simulink library "AeroLib"  (Simulink 6.0)
settings: Solver=ode45  SolverMode=SingleTasking  StartTime=0.0  StopTime=10.0  RelTol=1e-3
undefined symbols (not defined in the file): Aero, Ap, Atm, Control, Controls, Eng, Flight_cg, Flight_DamperON, Flight_delta_isa, Flight_DeltaSpiral, Flight_InertiaSelect, Flight_ixx, Flight_ixz, Flight_iyy, Flight_izz, Flight_latitude, Flight_LoiterLenght, Flight_LoiterMode, Flight_LoiterRadius, Flight_longitude, Flight_MaxTargetPoints, Flight_SensorsON, Flight_TimeStep, Flight_TowerWind_X, Flight_TowerWind_Y, Flight_TowerWind_Z, Flight_TowerWindON, Flight_Trimming, Flight_TurbON, Flight_weight, Flight_WindGustON, Flight_WindShearON, Flight_ycg, Flight_zcg, Geom, Lgear, Mass, PEG_CDwbnp, PEG_CLht, PEG_CLht_elev, PEG_CLwbnp, PEG_CMht, PEG_CMwbnp, PEG_CNbeta, PEG_CNr, PEG_CNrud, PEG_CRail, PEG_CRbeta, PEG_CRp, PEG_CRrud, PEG_CYbeta, PEG_CYrud, pow, Sensors
libraries: AeroLib x133, simulink3 x49, simulink x37, aerospace x11
(part 7 of 7)

== system AeroLib/Autopilot/Autopilot/Dampers/Pitch_Damper/Limit_Alpha_and_Speed ==
  TAS : Inport  Port=1  LatchInput=off
  Reset : Inport  Port=2  LatchInput=off
  From_Prop : Inport  Port=3  LatchInput=off
  Alpha : Inport  Port=4  LatchInput=off
  From_Inputs : Inport  Port=5  LatchInput=off
  Alpha Limit : Subsystem
  Bus Selector1 : BusSelector  DialogController=Simulink.DDGSource_Bus  OutputSignals=StopBooster
  Bus Selector2 : BusSelector  DialogController=Simulink.DDGSource_Bus  OutputSignals=IRU_TAS_kt
  Bus Selector3 : BusSelector  DialogController=Simulink.DDGSource_Bus  OutputSignals=BoosterON
  Logical Operator : Logic  Operator=OR
  Logical Operator1 : Logic  Operator=NOT
  Product1 : Product  SaturateOnIntegerOverflow=on  InputSameDT=on
  Saturation : Saturate  UpperLimit=5  LowerLimit=-5
  Speed_Limit : Subsystem
  Sum : Sum  Inputs=|++  SaturateOnIntegerOverflow=on  InputSameDT=on
  Elev_minSpeed : Outport
  wires:
  Saturation/1 -> Elev_minSpeed/1
  From_Prop/1 -> Bus Selector1/1
  Speed_Limit/1(Elev) -> Product1/1
  TAS/1 -> Bus Selector2/1
  Reset/1 -> Speed_Limit/2(Reset_In), Alpha Limit/2(Reset_In)
  Product1/1 -> Sum/1
  Alpha/1 -> Alpha Limit/1(Alpha)
  Alpha Limit/1(Elev) -> Sum/2
  Bus Selector2/1 -> Speed_Limit/1(TAS)  "<IRU_TAS_kt>"
  Sum/1 -> Saturation/1
  From_Inputs/1 -> Bus Selector3/1
  Bus Selector3/1 -> Logical Operator1/1  "<BoosterON>"
  Bus Selector1/1 -> Logical Operator/1  "<StopBooster>"
  Logical Operator1/1 -> Logical Operator/2
  Logical Operator/1 -> Product1/2

== system AeroLib/Autopilot/Autopilot/Dampers/Pitch_Damper/Pitch_damp ==
  From_INS : Inport  Port=1  LatchInput=off
  Bus Selector : BusSelector  DialogController=Simulink.DDGSource_Bus  OutputSignals=IRU_Q_degps,FSC_VD_mps
  Gain1 : Gain  Gain=Kq  SaturateOnIntegerOverflow=on
  Gain4 : Gain  Gain=Kd  SaturateOnIntegerOverflow=on
  Sum : Sum  SaturateOnIntegerOverflow=on  InputSameDT=on
  Elev_cmd : Outport
  wires:
  Gain4/1 -> Sum/2
  Bus Selector/2 -> Gain4/1  "<FSC_VD_mps>"
  Bus Selector/1 -> Gain1/1  "<IRU_Q_degps>"
  From_INS/1 -> Bus Selector/1
  Sum/1 -> Elev_cmd/1
  Gain1/1 -> Sum/1

== system AeroLib/Autopilot/Autopilot/Dampers/Roll_Damper/Phi Limit ==
  Reset_In : Inport  Port=1  LatchInput=off
  Phi : Inport  Port=2  LatchInput=off
  Abs : Abs  SaturateOnIntegerOverflow=on
  Bus Selector : BusSelector  DialogController=Simulink.DDGSource_Bus  OutputSignals=IRU_Phi_deg
  Constant : Constant  Value=0
  Gain : Gain  Gain=0.1  SaturateOnIntegerOverflow=on
  Stateless_HighPass : AeroLib/AMS_StatelessFilters/Stateless_HighPass
  Subsystem : Subsystem
  Sum2 : Sum  Inputs=|-+  SaturateOnIntegerOverflow=on  InputSameDT=on
  Switch : Switch  Threshold=Ap.Track.LimPhi+1  SaturateOnIntegerOverflow=on  InputSameDT=on
  Tau : Constant  Value=0.1
  Ail : Outport
  wires:
  Switch/1 -> Ail/1
  Subsystem/1(Ail_Com) -> Sum2/2
  Constant/1 -> Switch/3
  Bus Selector/1 -> Abs/1, Subsystem/1(Phi), Stateless_HighPass/2  "<IRU_Phi_deg>"
  Abs/1 -> Switch/2
  Gain/1 -> Sum2/1
  Sum2/1 -> Switch/1
  Stateless_HighPass/1 -> Gain/1
  Reset_In/1 -> Stateless_HighPass/1
  Tau/1 -> Stateless_HighPass/3
  Phi/1 -> Bus Selector/1

== system AeroLib/Autopilot/Autopilot/Dampers/Roll_Damper/Roll_damp ==
  From_Sen : Inport  Port=1  LatchInput=off
  Reset_In : Inport  Port=2  LatchInput=off
  Bus Selector : BusSelector  DialogController=Simulink.DDGSource_Bus  OutputSignals=IRU_P_degps,FSC_TrackMag_deg
  Damph_Gain : Gain  Gain=Kp  SaturateOnIntegerOverflow=on
  Damph_Gain1 : Gain  Gain=Kd  SaturateOnIntegerOverflow=on
  Deriv_Limit : Subsystem
  Stateless_HighPass : AeroLib/AMS_StatelessFilters/Stateless_HighPass
  Sum : Sum  SaturateOnIntegerOverflow=on  InputSameDT=on
  Tau : Constant  Value=0.1
  Ail_cmd : Outport
  wires:
  Deriv_Limit/1(Out) -> Damph_Gain1/1
  Sum/1 -> Ail_cmd/1
  Stateless_HighPass/1 -> Deriv_Limit/1(In)
  Damph_Gain1/1 -> Sum/2
  From_Sen/1 -> Bus Selector/1
  Bus Selector/1 -> Damph_Gain/1  "<IRU_P_degps>"
  Bus Selector/2 -> Stateless_HighPass/2  "<FSC_TrackMag_deg>"
  Damph_Gain/1 -> Sum/1
  Reset_In/1 -> Stateless_HighPass/1
  Tau/1 -> Stateless_HighPass/3

== system AeroLib/Autopilot/Autopilot/Dampers/Yaw_Damper/PID_Ny ==
  Err : Inport  Port=1  LatchInput=off
  From_Reset : Inport  Port=2  LatchInput=off
  IntGain : Gain  Gain=I  SaturateOnIntegerOverflow=on
  PID_Prop_Gamma : Gain  Gain=P  SaturateOnIntegerOverflow=on
  Stateless_HighPass : AeroLib/AMS_StatelessFilters/Stateless_HighPass
  Stateless_Integrator1 : AeroLib/AMS_StatelessFilters/Stateless_Integrator
  Sum : Sum  Inputs=+++  SaturateOnIntegerOverflow=on  InputSameDT=on
  Tau : Constant  Value=0.1
  Xo : Constant  Value=0
  Cmd : Outport  InitialOutput=0
  wires:
  Sum/1 -> Cmd/1
  Stateless_Integrator1/1 -> IntGain/1
  IntGain/1 -> Sum/2
  PID_Prop_Gamma/1 -> Sum/1
  Stateless_HighPass/1 -> Sum/3
  Err/1 -> Stateless_Integrator1/3, Stateless_HighPass/2, PID_Prop_Gamma/1
  Xo/1 -> Stateless_Integrator1/2
  From_Reset/1 -> Stateless_Integrator1/1, Stateless_HighPass/1
  Tau/1 -> Stateless_HighPass/3

== system AeroLib/Autopilot/Autopilot/Guidance/Loiter_modes/Last_point_data ==
  From_Sensors : Inport  Port=1  LatchInput=off
  Target_N : Inport  Port=2  LatchInput=off
  Bus Selector1 : BusSelector  DialogController=Simulink.DDGSource_Bus  OutputSignals=FSC_TrackMag_deg,FSC_Xdist_m,FSC_Ydist_m
  Demux : Demux  Outputs=3
  Fcn1 : Fcn  Expr=u(1) - u(2) == 1
  Mem : Memory  X0=[0 0 0]
  Memory : Memory
  Mux : Mux  Inputs=2
  Mux1 : Mux  Inputs=3
  Sw4 : Switch  Threshold=0.5  SaturateOnIntegerOverflow=on  InputSameDT=on
  deg-->rad : Gain  Gain=pi/180  SaturateOnIntegerOverflow=on
  LastX_m : Outport
  LastY_m : Outport  Port=2
  LastTrack_rad : Outport  Port=3
  wires:
  Demux/3 -> LastY_m/1
  Demux/2 -> LastX_m/1
  Demux/1 -> deg-->rad/1
  Mux1/1 -> Sw4/1
  Bus Selector1/3 -> Mux1/3  "<FSC_Ydist_m>"
  Bus Selector1/2 -> Mux1/2  "<FSC_Xdist_m>"
  Bus Selector1/1 -> Mux1/1  "<FSC_TrackMag_deg>"
  Target_N/1 -> Mux/1, Memory/1
  From_Sensors/1 -> Bus Selector1/1
  deg-->rad/1 -> LastTrack_rad/1
  Sw4/1 -> Mem/1
  Fcn1/1 -> Sw4/2
  Mem/1 -> Demux/1, Sw4/3
  Memory/1 -> Mux/2
  Mux/1 -> Fcn1/1

== system AeroLib/Autopilot/Autopilot/Guidance/Loiter_modes/Serpentine_Loiter_mode ==
  From_FSC : Inport  Port=1  LatchInput=off
  X_last : Inport  Port=2  LatchInput=off
  Y_last : Inport  Port=3  LatchInput=off
  Track_last : Inport  Port=4  LatchInput=off
  From_Reset : Inport  Port=5  LatchInput=off
  Bus Selector2 : BusSelector  DialogController=Simulink.DDGSource_Bus  OutputSignals=IRU_TAS_kt
  Constant : Constant
  Constant1 : Constant
  Counter_Point : AeroLib/Autopilot/Counter_Point  MinDist=Ap.Loiter.MinDist
  Fcn3 : Fcn  Expr=u+1
  Look-Up Table : Lookup  DialogController=Simulink.DDGSource  InputValues=[-360 -270 -180-eps -180+eps -90 0 90 180-eps 180+eps 270 360]  OutputValues=[0 90 180 -180 -90 0 90 180 -180 -90 0]  SaturateOnIntegerOverflow=on
  Memory_Dist : Memory  X0=1000000000
  Target_Errors : AeroLib/Autopilot/Target_Errors
  Terminator{,1..3} (4 alike) : Terminator
  Turn_Radius : Subsystem
  coord_serpent_or_lazy8 : Subsystem
  kt-->mps : Gain  Gain=0.5144444  SaturateOnIntegerOverflow=on
  Track_Err : Outport
  Point_N : Outport  Port=2
  wires:
  Turn_Radius/1(Track_Err) -> Track_Err/1
  Look-Up Table/1 -> Turn_Radius/1(Track_Error)
  coord_serpent_or_lazy8/2(X_target_m) -> Target_Errors/2
  coord_serpent_or_lazy8/1(Y_target_m) -> Target_Errors/1
  From_Reset/1 -> Counter_Point/2
  kt-->mps/1 -> Turn_Radius/2(TAS_mps)
  From_FSC/1 -> Bus Selector2/1, Target_Errors/4
  Y_last/1 -> coord_serpent_or_lazy8/3(Y_last)
  X_last/1 -> coord_serpent_or_lazy8/2(X_last)
  Track_last/1 -> coord_serpent_or_lazy8/1(track_last)
  Bus Selector2/1 -> kt-->mps/1  "<IRU_TAS_kt>"
  Target_Errors/3 -> Look-Up Table/1
  Counter_Point/1 -> Fcn3/1
  Memory_Dist/1 -> Counter_Point/1
  Fcn3/1 -> Point_N/1, coord_serpent_or_lazy8/4(Point_N)
  Target_Errors/2 -> Terminator/1
  Target_Errors/4 -> Terminator1/1
  Target_Errors/5 -> Terminator2/1
  Target_Errors/6 -> Terminator3/1
  Target_Errors/1 -> Memory_Dist/1
  Constant/1 -> Target_Errors/3
  Constant1/1 -> Target_Errors/5

== system AeroLib/Autopilot/Autopilot/Guidance/Loiter_modes/Spiral_and_circle_Loiter_mode ==
  LastTrack : Inport  Port=1  LatchInput=off
  From_FSC : Inport  Port=2  LatchInput=off
  From_Reset : Inport  Port=3  LatchInput=off
  Enable : EnablePort
  Bus Selector1 : BusSelector  DialogController=Simulink.DDGSource_Bus  OutputSignals=IRU_TAS_kt
  Bus Selector2 : BusSelector  DialogController=Simulink.DDGSource_Bus  OutputSignals=FSC_TrackMag_deg
  Constant2 : Constant  Orientation=left  Value=Flight_LoiterRadius
  Constant3 : Constant  Orientation=left  Value=Flight_DeltaSpiral
  Counter_Point : AeroLib/Autopilot/Counter_Point  MinDist=0.25
  Fcn1 : Fcn  Expr=abs( abs(u) - 90 )
  Fcn2 : Fcn  Orientation=left  Expr=u(2) + u(3)*u(1)
  Loiter_BankAngle : Fcn  Expr=atan(u(2)^2/(Atm.grav*u(1)))*180/pi/Ap.Track.err
  Mux1 : Mux  Orientation=left  Inputs=3
  Mux2 : Mux  Inputs=2
  Sum1 : Sum  Inputs=-+|  SaturateOnIntegerOverflow=on  InputSameDT=on
  kt-->mps : Gain  Gain=0.5144444  SaturateOnIntegerOverflow=on
  rad->deg : Gain  Gain=180/pi  SaturateOnIntegerOverflow=on
  Track_Err : Outport
  Point_N : Outport  Port=2
  wires:
  From_Reset/1 -> Counter_Point/2
  Constant3/1 -> Mux1/3
  Constant2/1 -> Mux1/2
  Mux1/1 -> Fcn2/1
  LastTrack/1 -> rad->deg/1
  Counter_Point/1 -> Mux1/1, Point_N/1
  Fcn2/1 -> Mux2/1
  kt-->mps/1 -> Mux2/2
  Bus Selector1/1 -> kt-->mps/1  "<IRU_TAS_kt>"
  Sum1/1 -> Fcn1/1
  Bus Selector2/1 -> Sum1/2  "<FSC_TrackMag_deg>"
  Loiter_BankAngle/1 -> Track_Err/1
  Mux2/1 -> Loiter_BankAngle/1
  From_FSC/1 -> Bus Selector1/1, Bus Selector2/1
  rad->deg/1 -> Sum1/1
  Fcn1/1 -> Counter_Point/1

== system AeroLib/Autopilot/Autopilot/Guidance/Loiter_modes/Subsystem ==
  Target_N : Inport  Port=1  LatchInput=off
  Constant1 : Constant  Value=Flight_LoiterMode
  Constant2 : Constant  Value=Flight_MaxTargetPoints
  Fcn1 : Fcn  Expr=u == 1
  Fcn2 : Fcn  Expr=u(1) >u(2)+0.5
  Logical Operator1 : Logic
  Mux : Mux  Inputs=2
  Enable_com : Outport
  wires:
  Target_N/1 -> Mux/1
  Constant2/1 -> Mux/2
  Mux/1 -> Fcn2/1
  Fcn1/1 -> Logical Operator1/2
  Constant1/1 -> Fcn1/1
  Logical Operator1/1 -> Enable_com/1
  Fcn2/1 -> Logical Operator1/1

== system AeroLib/Autopilot/Autopilot/Guidance/Target_Errors/AP_RATO ==
  FromSensor : Inport  Port=1  LatchInput=off
  From_Prop : Inport  Port=2  LatchInput=off
  From_Inputs : Inport  Port=3  LatchInput=off
  Bus Selector : BusSelector  DialogController=Simulink.DDGSource_Bus  OutputSignals=StopBooster
  Bus Selector1 : BusSelector  DialogController=Simulink.DDGSource_Bus  OutputSignals=IRU_TAS_kt,FSC_Altitude_ft
  Bus Selector2 : BusSelector  DialogController=Simulink.DDGSource_Bus  OutputSignals=BoosterON
  Fcn : Fcn  Expr=u(1) >= Ap.Booster.Vmin && u(2) >= Ap.Booster.Altmin
  Fcn1 : Fcn  Expr=1-u
  Mux2 : Mux  Inputs=2
  Product1 : Product  SaturateOnIntegerOverflow=on  InputSameDT=on
  Sum : Sum  Inputs=|++  SaturateOnIntegerOverflow=on  InputSameDT=on
  HoldAlt_ON : Outport
  wires:
  Fcn/1 -> Product1/2
  Bus Selector/1 -> Product1/1  "<StopBooster>"
  Bus Selector1/1 -> Mux2/1  "<IRU_TAS_kt>"
  Bus Selector1/2 -> Mux2/2  "<FSC_Altitude_ft>"
  Mux2/1 -> Fcn/1
  FromSensor/1 -> Bus Selector1/1
  From_Prop/1 -> Bus Selector/1
  From_Inputs/1 -> Bus Selector2/1
  Bus Selector2/1 -> Fcn1/1  "<BoosterON>"
  Product1/1 -> Sum/1
  Sum/1 -> HoldAlt_ON/1
  Fcn1/1 -> Sum/2

== system AeroLib/EquationsOfMotion/Equations_of_Motion/EQM Six-DOF/Geodetic_Frame_EQM/Longitude_Bound ==
  note: Latitude
      |
      | Longitude
  Lat Lon : Inport  Port=1  LatchInput=off
  Demux : Demux  Outputs=2
  Fcn2 : Fcn  Expr=u(1) + 360*u(2)
  Fcn3 : Fcn  Expr=u(1) - 360*u(2)
  Mux : Mux  Inputs=2
  Mux1 : Mux  Inputs=2
  Poles : Subsystem
  Subsystem : Subsystem
  Subsystem1 : Subsystem
  Switch2 : Switch  Threshold=-180  SaturateOnIntegerOverflow=on  InputSameDT=on
  Switch3 : Switch  Threshold=180  SaturateOnIntegerOverflow=on  InputSameDT=on
  Lon_deg : Outport
  Lat_deg : Outport  Port=2
  wires:
  Subsystem1/1(Out1) -> Mux1/2
  Mux1/1 -> Fcn2/1
  Subsystem/1(Out1) -> Mux/2
  Mux/1 -> Fcn3/1
  Lat Lon/1 -> Demux/1
  Demux/2 -> Poles/2(Longitude_deg)
  Demux/1 -> Lat_deg/1, Poles/1(Latitude_deg)
  Fcn2/1 -> Switch2/3
  Fcn3/1 -> Switch3/1
  Switch2/1 -> Switch3/2, Subsystem/1(In1), Mux/1, Switch3/3
  Switch3/1 -> Lon_deg/1
  Poles/1(LimLongitude_deg) -> Switch2/1, Subsystem1/1(In1), Mux1/1, Switch2/2

== system AeroLib/EquationsOfMotion/Equations_of_Motion/EQM Six-DOF/Geodetic_Frame_EQM/WGS 84 ==
  Latitude_rad : Inport  Port=1  LatchInput=off
  Altitude_m : Inport  Port=2  LatchInput=off
  Fcn : Fcn  Expr=(6378137+ u(2) )*(1-0.00669438)/(u(1)^1.5)
  Fcn1 : Fcn  Expr=(6378137+ u(2) )/sqrt(u(1))
  Fcn2 : Fcn  Expr=1-0.00669437999*(sin(u(1)))^2
  Fcn3 : Fcn  Expr=6378137 - 21385*sin(u(1))+u(2)
  Mux2 : Mux  Inputs=2
  Mux3 : Mux  Inputs=2
  RadOfCurv_ver_m : Outport
  GeogHight_m : Outport  Port=2
  RadOfCurv_mer_m : Outport  Port=3
  wires:
  Altitude_m/1 -> Mux2/2, Mux3/2
  Mux2/1 -> Fcn3/1
  Mux3/1 -> Fcn1/1, Fcn/1
  Latitude_rad/1 -> Mux2/1, Fcn2/1
  Fcn3/1 -> GeogHight_m/1
  Fcn1/1 -> RadOfCurv_ver_m/1
  Fcn/1 -> RadOfCurv_mer_m/1
  Fcn2/1 -> Mux3/1

== system AeroLib/EquationsOfMotion/Equations_of_Motion/EQM Six-DOF/Geodetic_Frame_EQM/Zero-->Eps ==
  In1 : Inport  Port=1  LatchInput=off
  Constant1 : Constant  Value=eps
  Fcn2 : Fcn  Expr=abs(u) > eps
  Product : Product  SaturateOnIntegerOverflow=on  InputSameDT=on
  Sign : Signum
  Switch : Switch  Threshold=0.5  SaturateOnIntegerOverflow=on  InputSameDT=on
  Out1 : Outport
  wires:
  Fcn2/1 -> Switch/2
  Sign/1 -> Product/1
  Constant1/1 -> Product/2
  Product/1 -> Switch/3
  Switch/1 -> Out1/1
  In1/1 -> Fcn2/1, Sign/1, Switch/1

== system AeroLib/EquationsOfMotion/Equations_of_Motion/EQM Six-DOF/Quaternion_Euler/Euler ==
  P Q R : Inport  Port=1  LatchInput=off
  Enable : EnablePort
  EQM Euler_Angles : Subsystem
  PHIang THETAang PSIang : Integrator
  Euler_Trim : Outport  InitialOutput=0
  wires:
  EQM Euler_Angles/1(phidot thetadot psidot) -> PHIang THETAang PSIang/1
  PHIang THETAang PSIang/1 -> EQM Euler_Angles/2(phi theta psi), Euler_Trim/1
  P Q R/1 -> EQM Euler_Angles/1(p q r)

== system AeroLib/EquationsOfMotion/Equations_of_Motion/EQM Six-DOF/Quaternion_Euler/Quaternion_Comp ==
  Flight_q : Inport  Port=1  LatchInput=off
  P Q R : Inport  Port=2  LatchInput=off
  Enable : EnablePort
  DeadZone : DeadZone  LowerValue=-eps  UpperValue=eps  SaturateOnIntegerOverflow=on
  QUA2EUL : AeroLib/CoordinateSystems/QUA2EUL
  Quaternion Normalize : Subsystem  mask(Quaternion Normalize){}
      mask help: qout = q/sqrt(q(1)^2+q(2)^2+q(3)^2+q(4)^2)
      mask init:
      | pos = get_param(gcb, 'Position');
      | width = pos(3) - pos(1); height = pos(4) - pos(2);
      | fontsize = get_param(gcb, 'fontsize');
      | scale=fontsize/10;
  Quaternion Derivative : Subsystem
      mask Display: disp('q = q1 + i*q2 + j*q3 + k*q4\n---------------------------------------------\nq1dot =-0.5*(q2*P + q3*Q + q4*R)\nq2dot = 0.5*(q1*P + q3*R -  q4*Q)\nq3dot = 0.5*(q1*Q + q3*P - q2*R)\nq4dot = 0.5*(q1*R + q2*Q - q3*P)')
  q1 q2 q3 q4 : Integrator  InitialConditionSource=external
  Euler  angles : Outport
  Quaternion : Outport  Port=2
  wires:
  DeadZone/1 -> q1 q2 q3 q4/1
  Quaternion Normalize/1(qnorm) -> QUA2EUL/1, Quaternion Derivative/2(q), Quaternion/1  "q1 q2 q3 q4"
  Flight_q/1 -> q1 q2 q3 q4/2
  Quaternion Derivative/1(q_dot) -> DeadZone/1
  q1 q2 q3 q4/1 -> Quaternion Normalize/1(q)
  P Q R/1 -> Quaternion Derivative/1(p q r)
  QUA2EUL/1 -> Euler  angles/1

== system AeroLib/EquationsOfMotion/Equations_of_Motion/EQM_Outputs/Inertilal Positions/Accelerations ==
  DCM : Inport  Port=1  LatchInput=off
  AG_b : Inport  Port=2  LatchInput=off
  Demux1 : Demux  Outputs=3
  Product : Product  Multiplication=Matrix(*)  SaturateOnIntegerOverflow=on  InputSameDT=on
  Xacc : Outport
  Yacc : Outport  Port=2
  Zacc : Outport  Port=3
  wires:
  Demux1/3 -> Zacc/1  "Zacc"
  Demux1/2 -> Yacc/1  "Yacc"
  Demux1/1 -> Xacc/1  "Xacc"
  AG_b/1 -> Product/2
  Product/1 -> Demux1/1  "AccI"
  DCM/1 -> Product/1

== system AeroLib/EquationsOfMotion/Equations_of_Motion/EQM_Outputs/Inertilal Positions/FlightPathVel ==
  AlongTrackAcc : Inport  Port=1  LatchInput=off
  Ang_rad : Inport  Port=2  LatchInput=off
  Zacc : Inport  Port=3  LatchInput=off
  Mux : Mux
  Trigonometric Function : Trigonometry
  Trigonometric Function1 : Trigonometry  Operator=cos
  Vert_acc : Fcn  Expr=- u / Atm.grav
  XcosA - YsinA : Fcn  Expr=(u(3)*u(2) - u(4)*u(1)) / Atm.grav
  AlongPathAcc_g : Outport
  VertAcc_g : Outport  Port=2
  wires:
  Vert_acc/1 -> VertAcc_g/1
  XcosA - YsinA/1 -> AlongPathAcc_g/1
  Mux/1 -> XcosA - YsinA/1
  Trigonometric Function/1 -> Mux/1
  Trigonometric Function1/1 -> Mux/2
  Zacc/1 -> Vert_acc/1, Mux/4
  AlongTrackAcc/1 -> Mux/3
  Ang_rad/1 -> Trigonometric Function1/1, Trigonometric Function/1

== system AeroLib/EquationsOfMotion/Equations_of_Motion/EQM_Outputs/Inertilal Positions/HeadingAcc ==
  Xacc : Inport  Port=1  LatchInput=off
  Yacc : Inport  Port=2  LatchInput=off
  Ang_rad : Inport  Port=3  LatchInput=off
  Mux : Mux
  Trigonometric Function : Trigonometry
  Trigonometric Function1 : Trigonometry  Operator=cos
  XcosA - YsinA : Fcn  Expr=(u(3)*u(2) - u(4)*u(1)) / Atm.grav
  YcosA + XsinA : Fcn  Expr=(u(4)*u(2) + u(3)*u(1)) / Atm.grav
  Along : Outport
  Cross : Outport  Port=2
  wires:
  YcosA + XsinA/1 -> Cross/1
  XcosA - YsinA/1 -> Along/1
  Mux/1 -> YcosA + XsinA/1, XcosA - YsinA/1
  Trigonometric Function/1 -> Mux/1
  Trigonometric Function1/1 -> Mux/2
  Yacc/1 -> Mux/4
  Xacc/1 -> Mux/3
  Ang_rad/1 -> Trigonometric Function1/1, Trigonometric Function/1

== system AeroLib/EquationsOfMotion/Equations_of_Motion/EQM_Outputs/Inertilal Positions/Positions ==
  Xe : Inport  Port=1  LatchInput=off
  Demux : Demux  Outputs=3
  Ground_Height : Constant  Value=0
  Sum : Sum  Inputs=|--  SaturateOnIntegerOverflow=on  InputSameDT=on
  m_to_ft : Gain  Gain=3.28083  SaturateOnIntegerOverflow=on
  Xdist : Outport  InitialOutput=0
  Ydist : Outport  Port=2  InitialOutput=0
  Hagl_m : Outport  Port=3  InitialOutput=0
  Hagl_ft : Outport  Port=4  InitialOutput=0
  wires:
  m_to_ft/1 -> Hagl_ft/1
  Sum/1 -> m_to_ft/1, Hagl_m/1
  Xe/1 -> Demux/1
  Demux/3 -> Sum/1
  Ground_Height/1 -> Sum/2
  Demux/2 -> Ydist/1
  Demux/1 -> Xdist/1

== system AeroLib/EquationsOfMotion/Equations_of_Motion/EQM_Outputs/Inertilal Positions/TrackAcc ==
  Ang_rad : Inport  Port=1  LatchInput=off
  Xdot : Inport  Port=2  LatchInput=off
  Ydot : Inport  Port=3  LatchInput=off
  Xacc : Inport  Port=4  LatchInput=off
  Yacc : Inport  Port=5  LatchInput=off
  Mux : Mux  Inputs=6
  Trigonometric Function : Trigonometry
  Trigonometric Function1 : Trigonometry  Operator=cos
  XcosA - YsinA : Fcn  Expr=(u(3)*u(2) - u(4)*u(1))
  YcosA + XsinA : Fcn  Expr=(u(4)*u(2) + u(3)*u(1))
  YcosA + XsinA1 : Fcn  Expr=(u(6)*u(2) + u(5)*u(1))
  AlongAcc : Outport
  CrossAcc : Outport  Port=2
  CrossTrackVel : Outport  Port=3
  wires:
  YcosA + XsinA1/1 -> CrossTrackVel/1
  Ydot/1 -> Mux/6
  Xdot/1 -> Mux/5
  YcosA + XsinA/1 -> CrossAcc/1
  XcosA - YsinA/1 -> AlongAcc/1
  Mux/1 -> YcosA + XsinA1/1, YcosA + XsinA/1, XcosA - YsinA/1
  Trigonometric Function/1 -> Mux/1
  Trigonometric Function1/1 -> Mux/2
  Yacc/1 -> Mux/4
  Xacc/1 -> Mux/3
  Ang_rad/1 -> Trigonometric Function1/1, Trigonometric Function/1

== system AeroLib/EquationsOfMotion/Equations_of_Motion/EQM_Outputs/Inertilal Positions/Velocities ==
  Vi : Inport  Port=1  LatchInput=off
  Fcn : Fcn  Expr=sqrt(u(1)*u(1)+u(2)*u(2))
  Fcn1 : Fcn  Expr=-u(3)
  Fcn2 : Fcn  Expr=u(1)
  Fcn3 : Fcn  Expr=-atan2(u(3),u(4))
  Fcn4 : Fcn  Expr=atan2(u(2),u(1))
  Fcn5 : Fcn  Expr=u(2)
  Mux1 : Mux  Inputs=2
  m/s_to_kt : Gain  Gain=1.943844  SaturateOnIntegerOverflow=on
  m/s_to_kt3 : Gain  Gain=196.8504  SaturateOnIntegerOverflow=on
  rad_to_deg : Gain  Gain=57.29578  SaturateOnIntegerOverflow=on
  rad_to_deg1 : Gain  Gain=57.29578  SaturateOnIntegerOverflow=on
  Hdot_mps : Outport  InitialOutput=0
  GroundSpeed_kt : Outport  Port=2  InitialOutput=0
  Gamma_deg : Outport  Port=3  InitialOutput=0
  Track_deg : Outport  Port=4  InitialOutput=0
  Hdot_ftpmin : Outport  Port=5  InitialOutput=0
  Track_rad : Outport  Port=6
  Xdot_mps : Outport  Port=7
  Ydot_mps : Outport  Port=8
  Gamma_rad : Outport  Port=9
  wires:
  Fcn3/1 -> rad_to_deg/1, Gamma_rad/1
  m/s_to_kt3/1 -> Hdot_ftpmin/1
  Fcn5/1 -> Ydot_mps/1
  Fcn2/1 -> Xdot_mps/1
  rad_to_deg1/1 -> Track_deg/1
  rad_to_deg/1 -> Gamma_deg/1
  m/s_to_kt/1 -> GroundSpeed_kt/1
  Fcn1/1 -> Hdot_mps/1, m/s_to_kt3/1
  Mux1/1 -> Fcn5/1, Fcn2/1, Fcn1/1, Fcn4/1, Fcn3/1
  Fcn/1 -> m/s_to_kt/1, Mux1/2  "GNS"
  Vi/1 -> Mux1/1, Fcn/1  "Ve"
  Fcn4/1 -> rad_to_deg1/1, Track_rad/1

== system AeroLib/GroundReactions/Landing_Gear/GHM Ground_Reactions/Reactions1/Inertial2Body ==
  FgLMG_I : Inport  Port=1  LatchInput=off
  FgNG_I : Inport  Port=2  LatchInput=off
  FgRMG_I : Inport  Port=3  LatchInput=off
  EulerRad : Inport  Port=4  LatchInput=off
  Demux : Demux  Outputs=3
  Ground2Body_LMG : Subsystem
  Ground2Body_NG : Subsystem
  Ground2Body_RMG : Subsystem
  Sum : Sum  Inputs=3  SaturateOnIntegerOverflow=on  InputSameDT=on
  Terminator : Terminator
  cos : Trigonometry  Operator=cos
  cos1 : Trigonometry  Operator=cos
  sin : Trigonometry
  sin1 : Trigonometry
  Fg_B : Outport
  FgLMG_B : Outport  Port=2
  FgNG_B : Outport  Port=3
  FgRMG_B : Outport  Port=4
  wires:
  Sum/1 -> Fg_B/1
  Ground2Body_RMG/1(Fg_B) -> Sum/3, FgRMG_B/1
  Ground2Body_NG/1(Fg_B) -> Sum/2, FgNG_B/1
  Ground2Body_LMG/1(Fg_B) -> Sum/1, FgLMG_B/1
  FgNG_I/1 -> Ground2Body_NG/1(Fb_I)
  FgLMG_I/1 -> Ground2Body_LMG/1(Fb_I)
  FgRMG_I/1 -> Ground2Body_RMG/1(Fb_I)
  cos/1 -> Ground2Body_NG/3(CosPhi), Ground2Body_LMG/3(CosPhi), Ground2Body_RMG/3(CosPhi)
  sin/1 -> Ground2Body_NG/2(SinPhi), Ground2Body_LMG/2(SinPhi), Ground2Body_RMG/2(SinPhi)
  cos1/1 -> Ground2Body_NG/5(CosThe), Ground2Body_LMG/5(CosThe), Ground2Body_RMG/5(CosThe)
  sin1/1 -> Ground2Body_NG/4(SinThe), Ground2Body_LMG/4(SinThe), Ground2Body_RMG/4(SinThe)
  Demux/3 -> Terminator/1  "psi"
  Demux/2 -> cos1/1, sin1/1  "theta"
  Demux/1 -> cos/1, sin/1  "phi"
  EulerRad/1 -> Demux/1

== system AeroLib/GroundReactions/Landing_Gear/GHM Ground_Reactions/Reactions1/NoseGearForces ==
  MUeNg : Inport  Port=1  LatchInput=off
  MUsNg : Inport  Port=2  LatchInput=off
  FstrNg : Inport  Port=3  LatchInput=off
  NoseWheelAng : Inport  Port=4  LatchInput=off
  Fcn : Fcn  Expr=u(3)*u(1) - u(4)*u(2)
  Fcn1 : Fcn  Expr=u(4)*u(1) + u(3)*u(2)
  Gain2 : Gain  Gain=-1  SaturateOnIntegerOverflow=on
  Mux : Mux
  Mux1 : Mux  Inputs=3
  Product1 : Product  SaturateOnIntegerOverflow=on  InputSameDT=on
  Product2 : Product  SaturateOnIntegerOverflow=on  InputSameDT=on
  Trigonometric Function : Trigonometry  Operator=cos
  Trigonometric Function1 : Trigonometry
  deg_to_rad : Gain  Gain=pi/180  SaturateOnIntegerOverflow=on
  FgearNG : Outport
  wires:
  NoseWheelAng/1 -> deg_to_rad/1
  Product1/1 -> Mux1/1
  Fcn/1 -> Product1/1  "Vx"
  Gain2/1 -> FgearNG/1
  FstrNg/1 -> Mux1/3, Product1/2, Product2/2
  Fcn1/1 -> Product2/1  "Vy"
  Product2/1 -> Mux1/2
  Mux/1 -> Fcn1/1, Fcn/1
  MUsNg/1 -> Mux/4
  MUeNg/1 -> Mux/3
  Trigonometric Function1/1 -> Mux/2
  Trigonometric Function/1 -> Mux/1
  Mux1/1 -> Gain2/1
  deg_to_rad/1 -> Trigonometric Function/1, Trigonometric Function1/1

== system AeroLib/GroundReactions/Landing_Gear/Left Main Gear Dynamics/Ground_Tire Friction/Friction Coeff ==
  Brake : Inport  Port=1  PortDimensions=1  LatchInput=off
  Ug : Inport  Port=2  PortDimensions=1  LatchInput=off
  Vg : Inport  Port=3  PortDimensions=1  LatchInput=off
  TireForce : Inport  Port=4  PortDimensions=1  LatchInput=off
  Constant : Constant  Value=.018
  Constant1 : Constant  Value=0.001
  Constant2 : Constant  Value=0.93
  Cpower : Constant  Value=110
  Fcn : Fcn  Expr=atan2(u(1),u(2))*180/pi
  Fcn2 : Fcn  Expr=2*u
  Fcn3 : Fcn  Expr=0.67-.0003*u
  Fcn4 : Fcn  Expr=u(3)+(u(1)-u(3))*u(2)
  MinMax1 : MinMax  Function=max  Inputs=2  SaturateOnIntegerOverflow=on  InputSameDT=on
  Mux : Mux  Inputs=2
  Mux2 : Mux  Inputs=3
  Product : Product  Inputs=**//  SaturateOnIntegerOverflow=on  InputSameDT=on
  Product1 : Product  SaturateOnIntegerOverflow=on  InputSameDT=on
  Saturation : Saturate  UpperLimit=1000  LowerLimit=1
  Sign : Signum
  MUside : Outport
  MUeff : Outport  Port=2
  wires:
  Mux/1 -> Fcn/1
  Vg/1 -> Mux/1
  Ug/1 -> Saturation/1, Sign/1
  Saturation/1 -> Mux/2, Fcn3/1
  TireForce/1 -> MinMax1/2
  Fcn/1 -> Product/2  "Beta"
  Constant2/1 -> Product/3
  MinMax1/1 -> Product/4
  Product/1 -> MUside/1  "MUside"
  Fcn3/1 -> Mux2/1  "MUdry"
  Brake/1 -> Mux2/2
  Mux2/1 -> Fcn4/1
  Constant/1 -> Mux2/3  "MuRoll"
  Constant1/1 -> MinMax1/1
  Cpower/1 -> Fcn2/1
  Fcn2/1 -> Product/1
  Fcn4/1 -> Product1/2
  Sign/1 -> Product1/1
  Product1/1 -> MUeff/1

== system AeroLib/GroundReactions/Landing_Gear/Nose Gear Dynamics/Ground_Tire Friction/Friction Coeff ==
  Ug : Inport  Port=1  PortDimensions=1  LatchInput=off
  Vg : Inport  Port=2  PortDimensions=1  LatchInput=off
  TireForce : Inport  Port=3  PortDimensions=1  LatchInput=off
  Constant1 : Constant  Value=0.001
  Constant2 : Constant  Value=0.93
  Constant4 : Constant  Value=.018
  Cpower : Constant  Value=110
  Fcn : Fcn  Expr=atan2(u(1),u(2))*180/pi
  Fcn2 : Fcn  Expr=2*u
  MinMax1 : MinMax  Function=max  Inputs=2  SaturateOnIntegerOverflow=on  InputSameDT=on
  Mux : Mux  Inputs=2
  Product : Product  Inputs=**//  SaturateOnIntegerOverflow=on  InputSameDT=on
  Product2 : Product  SaturateOnIntegerOverflow=on  InputSameDT=on
  Saturation : Saturate  UpperLimit=1000  LowerLimit=1
  Sign1 : Signum
  MUside : Outport
  MUeff : Outport  Port=2
  wires:
  Product2/1 -> MUeff/1
  Fcn2/1 -> Product/1
  Cpower/1 -> Fcn2/1
  Constant1/1 -> MinMax1/1
  Product/1 -> MUside/1  "MUside"
  MinMax1/1 -> Product/4
  Constant2/1 -> Product/3
  Fcn/1 -> Product/2  "Beta"
  TireForce/1 -> MinMax1/2
  Saturation/1 -> Mux/2
  Ug/1 -> Saturation/1, Sign1/1
  Vg/1 -> Mux/1
  Mux/1 -> Fcn/1
  Sign1/1 -> Product2/1
  Constant4/1 -> Product2/2  "MuRoll"

== system AeroLib/GroundReactions/Landing_Gear/Right Main Gear Dynamics/Ground_Tire Friction/Friction Coeff ==
  Brake : Inport  Port=1  PortDimensions=1  LatchInput=off
  Ug : Inport  Port=2  PortDimensions=1  LatchInput=off
  Vg : Inport  Port=3  PortDimensions=1  LatchInput=off
  TireForce : Inport  Port=4  PortDimensions=1  LatchInput=off
  Constant : Constant  Value=.018
  Constant1 : Constant  Value=0.001
  Constant2 : Constant  Value=0.93
  Cpower : Constant  Value=110
  Fcn : Fcn  Expr=atan2(u(1),u(2))*180/pi
  Fcn2 : Fcn  Expr=2*u
  Fcn3 : Fcn  Expr=0.67-.0003*u
  Fcn4 : Fcn  Expr=u(3)+(u(1)-u(3))*u(2)
  MinMax1 : MinMax  Function=max  Inputs=2  SaturateOnIntegerOverflow=on  InputSameDT=on
  Mux : Mux  Inputs=2
  Mux2 : Mux  Inputs=3
  Product : Product  Inputs=**//  SaturateOnIntegerOverflow=on  InputSameDT=on
  Product1 : Product  SaturateOnIntegerOverflow=on  InputSameDT=on
  Saturation : Saturate  UpperLimit=1000  LowerLimit=1
  Sign : Signum
  MUside : Outport
  MUeff : Outport  Port=2
  wires:
  Mux/1 -> Fcn/1
  Vg/1 -> Mux/1
  Ug/1 -> Saturation/1, Sign/1
  Saturation/1 -> Mux/2, Fcn3/1
  TireForce/1 -> MinMax1/2
  Fcn/1 -> Product/2  "Beta"
  Constant2/1 -> Product/3
  MinMax1/1 -> Product/4
  Product/1 -> MUside/1  "MUside"
  Fcn3/1 -> Mux2/1  "MUdry"
  Brake/1 -> Mux2/2
  Mux2/1 -> Fcn4/1
  Constant/1 -> Mux2/3  "MuRoll"
  Constant1/1 -> MinMax1/1
  Cpower/1 -> Fcn2/1
  Fcn2/1 -> Product/1
  Fcn4/1 -> Product1/2
  Sign/1 -> Product1/1
  Product1/1 -> MUeff/1

== system AeroLib/Sensors/Inertial_Reference_Unit/Accelerometers/Sensors/SensorsOFF ==
  Clock : Clock
      settings: Decimation=10
  Constant1 : Constant  Value=Flight_SensorsON
  Fcn : Fcn  Expr=u <= 0+eps
  or : Logic  Operator=OR
  or1 : Logic  Operator=NOT
  SensorsOFF : Outport
  wires:
  or1/1 -> or/1
  or/1 -> SensorsOFF/1
  Fcn/1 -> or/2
  Constant1/1 -> or1/1  "DT"
  Clock/1 -> Fcn/1

== system AeroLib/Autopilot/Autopilot/Dampers/Pitch_Damper/Limit_Alpha_and_Speed/Alpha Limit ==
  Alpha : Inport  Port=1  LatchInput=off
  Reset_In : Inport  Port=2  LatchInput=off
  Constant : Constant  Value=0
  Fcn : Fcn  Expr=-(u-Ap.Alt.MinAlpha)
  Gain2 : Gain  Gain=1.2  SaturateOnIntegerOverflow=on
  Stateless_HighPass1 : AeroLib/AMS_StatelessFilters/Stateless_HighPass
  Sum2 : Sum  Inputs=|-+  SaturateOnIntegerOverflow=on  InputSameDT=on
  Switch : Switch  Threshold=Ap.Alt.MinAlpha  SaturateOnIntegerOverflow=on  InputSameDT=on
  Tau : Constant  Value=0.1
  Elev : Outport
  wires:
  Tau/1 -> Stateless_HighPass1/3
  Reset_In/1 -> Stateless_HighPass1/1
  Switch/1 -> Elev/1
  Gain2/1 -> Sum2/1
  Fcn/1 -> Sum2/2
  Sum2/1 -> Switch/1
  Constant/1 -> Switch/3
  Alpha/1 -> Switch/2, Fcn/1, Stateless_HighPass1/2
  Stateless_HighPass1/1 -> Gain2/1

== system AeroLib/Autopilot/Autopilot/Dampers/Pitch_Damper/Limit_Alpha_and_Speed/Speed_Limit ==
  TAS : Inport  Port=1  LatchInput=off
  Reset_In : Inport  Port=2  LatchInput=off
  Constant : Constant  Value=0
  Fcn : Fcn  Expr=-(u-Ap.Alt.Vmin)
  Gain1 : Gain  Gain=-8  SaturateOnIntegerOverflow=on
  Gain2 : Gain  Gain=1.2  SaturateOnIntegerOverflow=on
  Stateless_HighPass : AeroLib/AMS_StatelessFilters/Stateless_HighPass
  Sum2 : Sum  Inputs=|-+  SaturateOnIntegerOverflow=on  InputSameDT=on
  Switch : Switch  Threshold=Ap.Alt.Vmin  SaturateOnIntegerOverflow=on  InputSameDT=on
  Tau : Constant  Value=0.1
  Elev : Outport
  wires:
  Gain1/1 -> Elev/1
  Sum2/1 -> Switch/3
  Constant/1 -> Switch/1
  Stateless_HighPass/1 -> Gain2/1
  TAS/1 -> Switch/2, Fcn/1, Stateless_HighPass/2
  Fcn/1 -> Sum2/2
  Gain2/1 -> Sum2/1
  Switch/1 -> Gain1/1
  Reset_In/1 -> Stateless_HighPass/1
  Tau/1 -> Stateless_HighPass/3

== system AeroLib/Autopilot/Autopilot/Dampers/Roll_Damper/Phi Limit/Subsystem ==
  Phi : Inport  Port=1  LatchInput=off
  Fcn1 : Fcn  Expr=u >= 0
  Fcn2 : Fcn  Expr=-( u - Ap.Track.LimPhi)*0.4
  Fcn3 : Fcn  Expr=-( u + Ap.Track.LimPhi)*0.4
  Switch1 : Switch  Threshold=0.5  SaturateOnIntegerOverflow=on  InputSameDT=on
  Ail_Com : Outport
  wires:
  Switch1/1 -> Ail_Com/1
  Phi/1 -> Fcn1/1, Fcn3/1, Fcn2/1
  Fcn3/1 -> Switch1/3
  Fcn2/1 -> Switch1/1
  Fcn1/1 -> Switch1/2

== system AeroLib/Autopilot/Autopilot/Dampers/Roll_Damper/Roll_damp/Deriv_Limit ==
  In : Inport  Port=1  LatchInput=off
  Constant1 : Constant  Value=Flight_TimeStep
  Mux : Mux  Inputs=2
  Product : Product  SaturateOnIntegerOverflow=on  InputSameDT=on
  limit : Fcn  Expr=abs(u(1)) < 15*u(2)
  Out : Outport
  wires:
  In/1 -> Product/1, Mux/1
  Product/1 -> Out/1
  limit/1 -> Product/2
  Mux/1 -> limit/1
  Constant1/1 -> Mux/2

== system AeroLib/Autopilot/Autopilot/Guidance/Loiter_modes/Serpentine_Loiter_mode/Turn_Radius ==
  Track_Error : Inport  Port=1  LatchInput=off
  TAS_mps : Inport  Port=2  LatchInput=off
  Abs : Abs  SaturateOnIntegerOverflow=on
  Constant : Constant  Value=Flight_LoiterRadius
  Fcn1 : Fcn  Expr=abs(u(1)) < abs(u(2))*1.1
  Loiter_BankAngle : Fcn  Expr=atan(u(2)^2/(Atm.grav*u(1)))*180/pi/Ap.Track.err
  Mux2 : Mux  Inputs=2
  Mux3 : Mux  Inputs=2
  Product : Product  SaturateOnIntegerOverflow=on  InputSameDT=on
  Sign : Signum
  Switch : Switch  Threshold=0.5  SaturateOnIntegerOverflow=on  InputSameDT=on
  Track_Err : Outport
  wires:
  TAS_mps/1 -> Mux2/2
  Constant/1 -> Mux2/1
  Product/1 -> Switch/3
  Sign/1 -> Product/1
  Abs/1 -> Mux3/2, Product/2
  Loiter_BankAngle/1 -> Abs/1
  Switch/1 -> Track_Err/1
  Mux3/1 -> Fcn1/1
  Fcn1/1 -> Switch/2
  Mux2/1 -> Loiter_BankAngle/1
  Track_Error/1 -> Mux3/1, Sign/1, Switch/1

== system AeroLib/Autopilot/Autopilot/Guidance/Loiter_modes/Serpentine_Loiter_mode/coord_serpent_or_lazy8 ==
  track_last : Inport  Port=1  LatchInput=off
  X_last : Inport  Port=2  LatchInput=off
  Y_last : Inport  Port=3  LatchInput=off
  Point_N : Inport  Port=4  LatchInput=off
  Constant1 : Constant  Value=Flight_LoiterMode
  Demux : Demux  Outputs=2
  Gain1 : Gain  Gain=-1  SaturateOnIntegerOverflow=on
  LazyEight_Coor : Subsystem
  Mux1 : Mux  Inputs=2
  Product : Product  Multiplication=Matrix(*)  SaturateOnIntegerOverflow=on  InputSameDT=on
  Reshape : simulink/Math Operations/Reshape  OutputDimensionality=Row vector  OutputDimensions=[1,1]
  Serpentine_Coor : Subsystem
  Sum : Sum  Inputs=|++  SaturateOnIntegerOverflow=on  InputSameDT=on
  Switch : Switch  Threshold=2.5  SaturateOnIntegerOverflow=on  InputSameDT=on
  turn_transform : Subsystem
  Y_target_m : Outport
  X_target_m : Outport  Port=2
  wires:
  Constant1/1 -> Switch/2
  LazyEight_Coor/1(XY) -> Switch/1
  Switch/1 -> Reshape/1
  Serpentine_Coor/1(XY) -> Switch/3
  Gain1/1 -> turn_transform/1(Track_rad)
  Reshape/1 -> Product/1
  turn_transform/1(MatrixTransform) -> Product/2
  Y_last/1 -> Mux1/2
  X_last/1 -> Mux1/1
  Demux/2 -> Y_target_m/1
  Demux/1 -> X_target_m/1
  track_last/1 -> Gain1/1
  Sum/1 -> Demux/1
  Point_N/1 -> Serpentine_Coor/1(Point_N), LazyEight_Coor/1(Point_N)
  Product/1 -> Sum/1
  Mux1/1 -> Sum/2

== system AeroLib/EquationsOfMotion/Equations_of_Motion/EQM Six-DOF/Geodetic_Frame_EQM/Longitude_Bound/Poles ==
  Latitude_deg : Inport  Port=1  LatchInput=off
  Longitude_deg : Inport  Port=2  LatchInput=off
  Fcn1 : Fcn  Expr=abs(abs(u ) - 90) < 0.00001
  Fcn2 : Fcn  Expr=u(1)+180*u(2)
  Memory : Memory
  Mux : Mux  Inputs=2
  Sum : Sum  Inputs=|++  SaturateOnIntegerOverflow=on  InputSameDT=on
  Switch2 : Switch  Threshold=0.5  SaturateOnIntegerOverflow=on  InputSameDT=on
  LimLongitude_deg : Outport
  wires:
  Mux/1 -> Fcn2/1
  Fcn2/1 -> Switch2/1
  Fcn1/1 -> Sum/1
  Sum/1 -> Memory/1
  Memory/1 -> Sum/2, Switch2/2, Mux/2
  Longitude_deg/1 -> Switch2/3, Mux/1
  Switch2/1 -> LimLongitude_deg/1
  Latitude_deg/1 -> Fcn1/1

== system AeroLib/EquationsOfMotion/Equations_of_Motion/EQM Six-DOF/Geodetic_Frame_EQM/Longitude_Bound/Subsystem ==
  In1 : Inport  Port=1  LatchInput=off
  Constant : Constant
  Fcn1 : Fcn  Expr=u/360
  MinMax : MinMax  Function=max  Inputs=2  SaturateOnIntegerOverflow=on  InputSameDT=on
  Rounding Function : Rounding  Operator=round
  Out1 : Outport
  wires:
  Rounding Function/1 -> Out1/1
  In1/1 -> Fcn1/1
  Fcn1/1 -> MinMax/1
  MinMax/1 -> Rounding Function/1
  Constant/1 -> MinMax/2

== system AeroLib/EquationsOfMotion/Equations_of_Motion/EQM Six-DOF/Geodetic_Frame_EQM/Longitude_Bound/Subsystem1 ==
  In1 : Inport  Port=1  LatchInput=off
  Constant : Constant
  Fcn1 : Fcn  Expr=abs(u/360)
  MinMax : MinMax  Function=max  Inputs=2  SaturateOnIntegerOverflow=on  InputSameDT=on
  Rounding Function : Rounding  Operator=round
  Out1 : Outport
  wires:
  Constant/1 -> MinMax/2
  MinMax/1 -> Rounding Function/1
  Fcn1/1 -> MinMax/1
  In1/1 -> Fcn1/1
  Rounding Function/1 -> Out1/1

== system AeroLib/EquationsOfMotion/Equations_of_Motion/EQM Six-DOF/Quaternion_Euler/Euler/EQM Euler_Angles ==
  p q r : Inport  Port=1  LatchInput=off
  phi theta psi : Inport  Port=2  LatchInput=off
  Mux1 : Mux  Inputs=[3 3]
  Mux2 : Mux  Inputs=3
  phidot : Fcn  Expr=u[1]+u[2]*sin(u[4])*tan(u[5])+u[3]*cos(u[4])*tan(u[5])
  psidot : Fcn  Expr=u[2]*sin(u[4])/cos(u[5])+u[3]*cos(u[4])/cos(u[5])
  thetadot : Fcn  Expr=u[2]*cos(u[4])-u[3]*sin(u[4])
  phidot thetadot psidot : Outport  InitialOutput=0
  wires:
  phidot/1 -> Mux2/1
  thetadot/1 -> Mux2/2
  psidot/1 -> Mux2/3
  phi theta psi/1 -> Mux1/2
  p q r/1 -> Mux1/1
  Mux1/1 -> phidot/1, psidot/1, thetadot/1
  Mux2/1 -> phidot thetadot psidot/1

== system AeroLib/EquationsOfMotion/Equations_of_Motion/EQM Six-DOF/Quaternion_Euler/Quaternion_Comp/Quaternion Normalize ==
  q : Inport  Port=1  PortDimensions=4  LatchInput=off
  Product : Product  Inputs=*/  SaturateOnIntegerOverflow=on  InputSameDT=on
  Square : Math  Operator=square  SaturateOnIntegerOverflow=on
  Square Root : Math  Operator=sqrt  SaturateOnIntegerOverflow=on
  Sum : Sum  Inputs=1  SaturateOnIntegerOverflow=on  InputSameDT=on
  qnorm : Outport  InitialOutput=0
  wires:
  Product/1 -> qnorm/1
  Square Root/1 -> Product/2
  q/1 -> Product/1, Square/1
  Square/1 -> Sum/1
  Sum/1 -> Square Root/1

== system AeroLib/EquationsOfMotion/Equations_of_Motion/EQM Six-DOF/Quaternion_Euler/Quaternion_Comp/Quaternion Derivative ==
  p q r : Inport  Port=1  LatchInput=off
  q : Inport  Port=2  LatchInput=off
  Mux1 : Mux  Inputs=2
  Mux2 : Mux
  q1dot : Fcn  Expr=-0.5 * ( u[5]*u[1]+u[6]*u[2]+u[7]*u[3] )
  q2dot : Fcn  Expr=0.5 * ( u[4]*u[1]+u[6]*u[3]-u[7]*u[2] )
  q3dot : Fcn  Expr=0.5 * ( u[4]*u[2]+u[7]*u[1]-u[5]*u[3] )
  q4dot : Fcn  Expr=0.5 * ( u[4]*u[3]+u[5]*u[2]-u[6]*u[1] )
  q_dot : Outport  InitialOutput=0
  wires:
  q/1 -> Mux1/2
  q4dot/1 -> Mux2/4
  Mux1/1 -> q4dot/1, q3dot/1, q2dot/1, q1dot/1
  q3dot/1 -> Mux2/3
  q2dot/1 -> Mux2/2
  q1dot/1 -> Mux2/1
  p q r/1 -> Mux1/1
  Mux2/1 -> q_dot/1

== system AeroLib/GroundReactions/Landing_Gear/GHM Ground_Reactions/Reactions1/Inertial2Body/Ground2Body_LMG ==
  Fb_I : Inport  Port=1  LatchInput=off
  SinPhi : Inport  Port=2  LatchInput=off
  CosPhi : Inport  Port=3  LatchInput=off
  SinThe : Inport  Port=4  LatchInput=off
  CosThe : Inport  Port=5  LatchInput=off
  Demux : Demux  Outputs=3
  Mux1 : Mux  Inputs=7
  Mux2 : Mux  Inputs=2
  Mux3 : Mux  Inputs=3
  Xb : Fcn  Expr=u(1)*u(7) - u(3)*u(6)
  Yb : Fcn  Expr=u(2)*u(5) + u(8)*u(4)
  Zb : Fcn  Expr=u(8)*u(5) - u(2)*u(4)
  Zbp : Fcn  Expr=u(3)*u(7) + u(1)*u(6)
  Fg_B : Outport
  wires:
  Fb_I/1 -> Demux/1
  Mux3/1 -> Fg_B/1
  Zb/1 -> Mux3/3
  Yb/1 -> Mux3/2
  Xb/1 -> Mux3/1
  Mux2/1 -> Zb/1, Yb/1
  Zbp/1 -> Mux2/2  "Zbp_u(8)"
  Demux/2 -> Mux1/2  "YI_u(2)"
  Mux1/1 -> Mux2/1, Xb/1, Zbp/1
  Demux/3 -> Mux1/3  "ZI_u(3)"
  Demux/1 -> Mux1/1  "XI_u(1)"
  CosThe/1 -> Mux1/7  "cthe_u(7)"
  SinThe/1 -> Mux1/6  "sthe_u(6)"
  CosPhi/1 -> Mux1/5  "cphi_u(5)"
  SinPhi/1 -> Mux1/4  "sphi_u(4)"

== system AeroLib/GroundReactions/Landing_Gear/GHM Ground_Reactions/Reactions1/Inertial2Body/Ground2Body_NG ==
  Fb_I : Inport  Port=1  LatchInput=off
  SinPhi : Inport  Port=2  LatchInput=off
  CosPhi : Inport  Port=3  LatchInput=off
  SinThe : Inport  Port=4  LatchInput=off
  CosThe : Inport  Port=5  LatchInput=off
  Demux : Demux  Outputs=3
  Mux1 : Mux  Inputs=7
  Mux2 : Mux  Inputs=2
  Mux3 : Mux  Inputs=3
  Xb : Fcn  Expr=u(1)*u(7) - u(3)*u(6)
  Yb : Fcn  Expr=u(2)*u(5) + u(8)*u(4)
  Zb : Fcn  Expr=u(8)*u(5) - u(2)*u(4)
  Zbp : Fcn  Expr=u(3)*u(7) + u(1)*u(6)
  Fg_B : Outport
  wires:
  SinPhi/1 -> Mux1/4  "sphi_u(4)"
  CosPhi/1 -> Mux1/5  "cphi_u(5)"
  SinThe/1 -> Mux1/6  "sthe_u(6)"
  CosThe/1 -> Mux1/7  "cthe_u(7)"
  Demux/1 -> Mux1/1  "XI_u(1)"
  Demux/3 -> Mux1/3  "ZI_u(3)"
  Mux1/1 -> Zbp/1, Xb/1, Mux2/1
  Demux/2 -> Mux1/2  "YI_u(2)"
  Zbp/1 -> Mux2/2  "Zbp_u(8)"
  Mux2/1 -> Yb/1, Zb/1
  Xb/1 -> Mux3/1
  Yb/1 -> Mux3/2
  Zb/1 -> Mux3/3
  Mux3/1 -> Fg_B/1
  Fb_I/1 -> Demux/1

== system AeroLib/GroundReactions/Landing_Gear/GHM Ground_Reactions/Reactions1/Inertial2Body/Ground2Body_RMG ==
  Fb_I : Inport  Port=1  LatchInput=off
  SinPhi : Inport  Port=2  LatchInput=off
  CosPhi : Inport  Port=3  LatchInput=off
  SinThe : Inport  Port=4  LatchInput=off
  CosThe : Inport  Port=5  LatchInput=off
  Demux : Demux  Outputs=3
  Mux1 : Mux  Inputs=7
  Mux2 : Mux  Inputs=2
  Mux3 : Mux  Inputs=3
  Xb : Fcn  Expr=u(1)*u(7) - u(3)*u(6)
  Yb : Fcn  Expr=u(2)*u(5) + u(8)*u(4)
  Zb : Fcn  Expr=u(8)*u(5) - u(2)*u(4)
  Zbp : Fcn  Expr=u(3)*u(7) + u(1)*u(6)
  Fg_B : Outport
  wires:
  Fb_I/1 -> Demux/1
  Mux3/1 -> Fg_B/1
  Zb/1 -> Mux3/3
  Yb/1 -> Mux3/2
  Xb/1 -> Mux3/1
  Mux2/1 -> Zb/1, Yb/1
  Zbp/1 -> Mux2/2  "Zbp_u(8)"
  Demux/2 -> Mux1/2  "YI_u(2)"
  Mux1/1 -> Mux2/1, Xb/1, Zbp/1
  Demux/3 -> Mux1/3  "ZI_u(3)"
  Demux/1 -> Mux1/1  "XI_u(1)"
  CosThe/1 -> Mux1/7  "cthe_u(7)"
  SinThe/1 -> Mux1/6  "sthe_u(6)"
  CosPhi/1 -> Mux1/5  "cphi_u(5)"
  SinPhi/1 -> Mux1/4  "sphi_u(4)"

== system AeroLib/Autopilot/Autopilot/Guidance/Loiter_modes/Serpentine_Loiter_mode/coord_serpent_or_lazy8/LazyEight_Coor ==
  Point_N : Inport  Port=1  LatchInput=off
  Mux3 : Mux  Inputs=2
  X_axis : Subsystem
  Y_Axis : Subsystem
  XY : Outport
  wires:
  Mux3/1 -> XY/1
  Point_N/1 -> Y_Axis/1(Point_N), X_axis/1(Point_N)
  Y_Axis/1(Y) -> Mux3/2
  X_axis/1(X) -> Mux3/1

== system AeroLib/Autopilot/Autopilot/Guidance/Loiter_modes/Serpentine_Loiter_mode/coord_serpent_or_lazy8/Serpentine_Coor ==
  Point_N : Inport  Port=1  LatchInput=off
  Constant2 : Constant  Value=Flight_LoiterRadius
  Constant3 : Constant  Value=Flight_LoiterLenght
  Memory : Memory
  Mux1 : Mux  Inputs=2
  Mux3 : Mux  Inputs=2
  Mux4 : Mux  Inputs=2
  Sum1 : Sum  Inputs=|++  SaturateOnIntegerOverflow=on  InputSameDT=on
  X : Fcn  Expr=u(2)*(u(1)-1)
  Y : Fcn  Expr=-(u(2)/2)*(-1)^u(1)
  XY : Outport
  wires:
  Mux4/1 -> XY/1
  Constant3/1 -> Mux3/2
  Mux3/1 -> Y/1
  Constant2/1 -> Mux1/2
  Mux1/1 -> X/1
  Y/1 -> Mux4/2
  X/1 -> Mux4/1
  Sum1/1 -> Mux1/1
  Memory/1 -> Sum1/2
  Point_N/1 -> Sum1/1, Mux3/1, Memory/1

== system AeroLib/Autopilot/Autopilot/Guidance/Loiter_modes/Serpentine_Loiter_mode/coord_serpent_or_lazy8/turn_transform ==
  Track_rad : Inport  Port=1  LatchInput=off
  Gain2 : Gain  Gain=-1  SaturateOnIntegerOverflow=on
  Mux2 : Mux
  Reshape : simulink/Math Operations/Reshape  OutputDimensionality=Customize  OutputDimensions=[2,2]
  Trigonometric Function : Trigonometry
  Trigonometric Function1 : Trigonometry  Operator=cos
  Trigonometric Function2 : Trigonometry
  Trigonometric Function3 : Trigonometry  Operator=cos
  MatrixTransform : Outport
  wires:
  Gain2/1 -> Trigonometric Function2/1
  Trigonometric Function2/1 -> Mux2/3
  Reshape/1 -> MatrixTransform/1
  Track_rad/1 -> Gain2/1, Trigonometric Function3/1, Trigonometric Function/1, Trigonometric Function1/1
  Mux2/1 -> Reshape/1
  Trigonometric Function3/1 -> Mux2/4
  Trigonometric Function/1 -> Mux2/2
  Trigonometric Function1/1 -> Mux2/1

== system AeroLib/Autopilot/Autopilot/Guidance/Loiter_modes/Serpentine_Loiter_mode/coord_serpent_or_lazy8/LazyEight_Coor/X_axis ==
  Point_N : Inport  Port=1  LatchInput=off
  Constant3 : Constant  Value=Flight_LoiterRadius
  Constant4 : Constant  Value=0
  Fcn : Fcn  Expr=floor(u/2) - u/2 == 0
  Gain : Gain  Gain=2  SaturateOnIntegerOverflow=on
  Switch2 : Switch  Threshold=0.5  SaturateOnIntegerOverflow=on  InputSameDT=on
  X : Outport
  wires:
  Gain/1 -> Switch2/1
  Point_N/1 -> Fcn/1
  Switch2/1 -> X/1
  Constant4/1 -> Switch2/3
  Constant3/1 -> Gain/1
  Fcn/1 -> Switch2/2

== system AeroLib/Autopilot/Autopilot/Guidance/Loiter_modes/Serpentine_Loiter_mode/coord_serpent_or_lazy8/LazyEight_Coor/Y_Axis ==
  Point_N : Inport  Port=1  LatchInput=off
  Fcn1 : Fcn  Expr=u > 4.5
  Fcn2 : Fcn  Expr=u > 4.5
  Fcn3 : Fcn  Expr=u-4
  Fcn5 : Fcn  Expr=u-4
  Gain : Gain  Gain=0.5  SaturateOnIntegerOverflow=on
  Selector : Selector  ElementSrc=External  Elements=[2 ]  RowSrc=External  Rows=5  Columns=-1  InputPortWidth=4
  Switch : Switch  Threshold=0.5  SaturateOnIntegerOverflow=on  InputSameDT=on
  Switch1 : Switch  Threshold=0.5  SaturateOnIntegerOverflow=on  InputSameDT=on
  Y_Coordinat : Subsystem
  Y : Outport
  wires:
  Gain/1 -> Selector/1
  Selector/1 -> Y/1
  Switch1/1 -> Selector/2
  Y_Coordinat/1(Y) -> Gain/1
  Fcn5/1 -> Switch1/1
  Fcn2/1 -> Switch1/2
  Switch/1 -> Fcn5/1, Switch1/3, Fcn2/1
  Fcn3/1 -> Switch/1
  Point_N/1 -> Fcn3/1, Switch/3, Fcn1/1
  Fcn1/1 -> Switch/2

== system AeroLib/Autopilot/Autopilot/Guidance/Loiter_modes/Serpentine_Loiter_mode/coord_serpent_or_lazy8/LazyEight_Coor/Y_Axis/Y_Coordinat ==
  Constant{1..2,4..5} (4 alike) : Constant  Value=Flight_LoiterLenght
  Gain : Gain  Gain=-1  SaturateOnIntegerOverflow=on
  Gain1 : Gain  Gain=-1  SaturateOnIntegerOverflow=on
  Mux : Mux
  Y : Outport
  wires:
  Gain1/1 -> Mux/4
  Gain/1 -> Mux/3
  Mux/1 -> Y/1
  Constant1/1 -> Mux/1
  Constant2/1 -> Mux/2
  Constant4/1 -> Gain/1
  Constant5/1 -> Gain1/1
